simulink subsystem "wheelSpeed"  (R2022b)
settings: Solver=VariableStepAuto  StartTime=0.0  StopTime=10.0  RelTol=1e-3
libraries: wheels x4
settings Model: Creator=serga  LastModifiedBy=serga

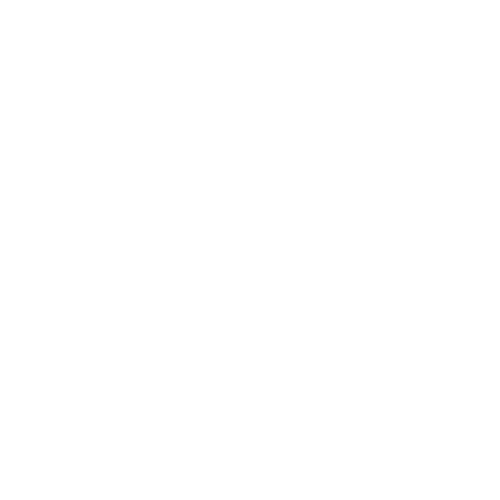
[thumbnail: Simulink's stored preview of the top-level diagram]
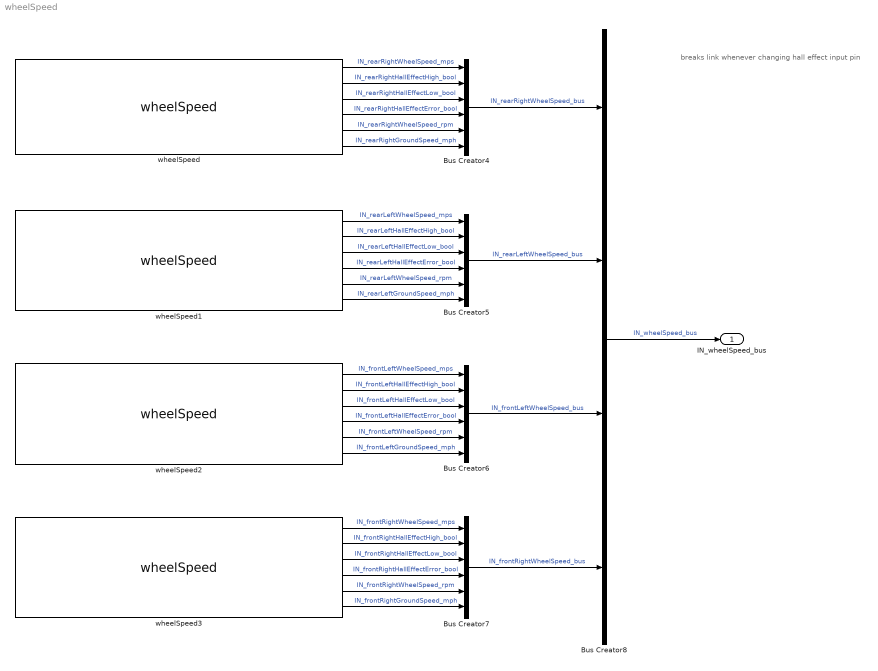
== system wheelSpeed ==
  note: breaks link whenever changing hall effect input pin
  Bus Creator{4..7} (4 alike) : BusCreator  Inputs=6
  Bus Creator8 : BusCreator  Inputs=4
  wheelSpeed : wheels/wheelSpeed  pos='RR'
  wheelSpeed1 : wheels/wheelSpeed  pos='RL'
  wheelSpeed2 : wheels/wheelSpeed  pos='FL'
  wheelSpeed3 : wheels/wheelSpeed  pos='FR'
  IN_wheelSpeed_bus : Outport
  wires:
  wheelSpeed1/3 -> Bus Creator5/3  "IN_rearLeftHallEffectLow_bool"
  wheelSpeed2/5 -> Bus Creator6/5  "IN_frontLeftWheelSpeed_rpm"
  wheelSpeed1/2 -> Bus Creator5/2  "IN_rearLeftHallEffectHigh_bool"
  wheelSpeed3/3 -> Bus Creator7/3  "IN_frontRightHallEffectLow_bool"
  wheelSpeed/1 -> Bus Creator4/1  "IN_rearRightWheelSpeed_mps"
  Bus Creator6/1 -> Bus Creator8/3  "IN_frontLeftWheelSpeed_bus"
  wheelSpeed1/1 -> Bus Creator5/1  "IN_rearLeftWheelSpeed_mps"
  wheelSpeed/5 -> Bus Creator4/5  "IN_rearRightWheelSpeed_rpm"
  Bus Creator5/1 -> Bus Creator8/2  "IN_rearLeftWheelSpeed_bus"
  wheelSpeed3/2 -> Bus Creator7/2  "IN_frontRightHallEffectHigh_bool"
  wheelSpeed3/6 -> Bus Creator7/6  "IN_frontRightGroundSpeed_mph"
  wheelSpeed2/3 -> Bus Creator6/3  "IN_frontLeftHallEffectLow_bool"
  wheelSpeed2/1 -> Bus Creator6/1  "IN_frontLeftWheelSpeed_mps"
  wheelSpeed1/5 -> Bus Creator5/5  "IN_rearLeftWheelSpeed_rpm"
  Bus Creator8/1 -> IN_wheelSpeed_bus/1  "IN_wheelSpeed_bus"
  wheelSpeed2/2 -> Bus Creator6/2  "IN_frontLeftHallEffectHigh_bool"
  wheelSpeed1/4 -> Bus Creator5/4  "IN_rearLeftHallEffectError_bool"
  wheelSpeed3/5 -> Bus Creator7/5  "IN_frontRightWheelSpeed_rpm"
  wheelSpeed/3 -> Bus Creator4/3  "IN_rearRightHallEffectLow_bool"
  Bus Creator7/1 -> Bus Creator8/4  "IN_frontRightWheelSpeed_bus"
  wheelSpeed/4 -> Bus Creator4/4  "IN_rearRightHallEffectError_bool"
  wheelSpeed2/6 -> Bus Creator6/6  "IN_frontLeftGroundSpeed_mph"
  wheelSpeed1/6 -> Bus Creator5/6  "IN_rearLeftGroundSpeed_mph"
  wheelSpeed3/4 -> Bus Creator7/4  "IN_frontRightHallEffectError_bool"
  wheelSpeed2/4 -> Bus Creator6/4  "IN_frontLeftHallEffectError_bool"
  wheelSpeed/6 -> Bus Creator4/6  "IN_rearRightGroundSpeed_mph"
  Bus Creator4/1 -> Bus Creator8/1  "IN_rearRightWheelSpeed_bus"
  wheelSpeed3/1 -> Bus Creator7/1  "IN_frontRightWheelSpeed_mps"
  wheelSpeed/2 -> Bus Creator4/2  "IN_rearRightHallEffectHigh_bool"
